simulink model "ThrottleAirMassFlow"  (R2025b)
settings: Solver=FixedStepAuto  StartTime=0.0  StopTime=200  FixedStep=0.001  RelTol=1e-3
undefined symbols (not defined in the file): R
settings Model: Creator=khanh  LastModifiedBy=khanh

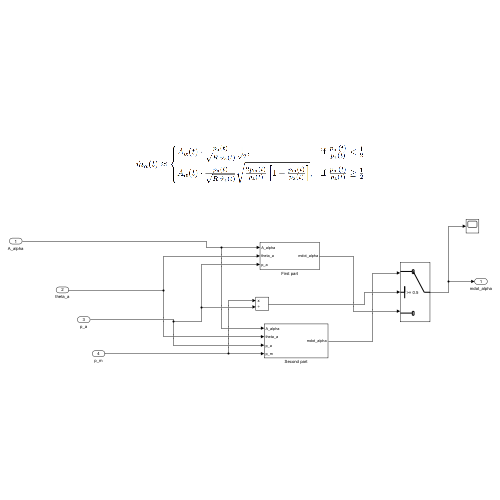
[thumbnail: Simulink's stored preview of the top-level diagram]
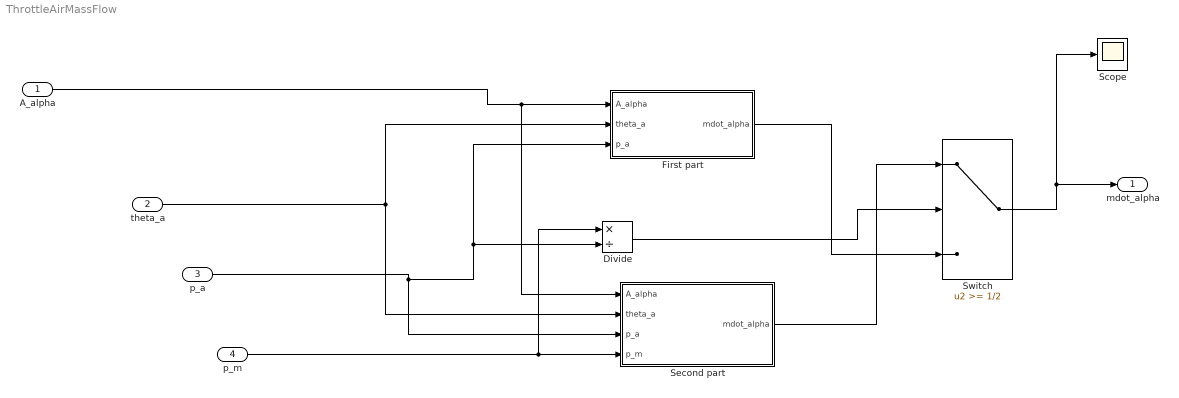
== system ThrottleAirMassFlow ==
  A_alpha : Inport
  theta_a : Inport  Port=2
  p_a : Inport  Port=3
  p_m : Inport  Port=4
  Divide : Product  Inputs=*/
  First part : Subsystem
  Scope : Scope
      settings: ActiveDisplayYMinimum=154.82054401919723  ActiveDisplayYMaximum=232.27112620786752
  "Second part " : Subsystem
  Switch : Switch  Threshold=1/2  SaturateOnIntegerOverflow=off  InputSameDT=off
  mdot_alpha : Outport
  wires:
  theta_a/1 -> "Second part "/2(theta_a), First part/2(theta_a)
  p_a/1 -> "Second part "/3(p_a), First part/3(p_a), Divide/2
  p_m/1 -> "Second part "/4(p_m), Divide/1
  Divide/1 -> Switch/2
  First part/1(mdot_alpha) -> Switch/3
  Switch/1 -> Scope/1, mdot_alpha/1
  "Second part "/1(mdot_alpha) -> Switch/1
  A_alpha/1 -> "Second part "/1(A_alpha), First part/1(A_alpha)

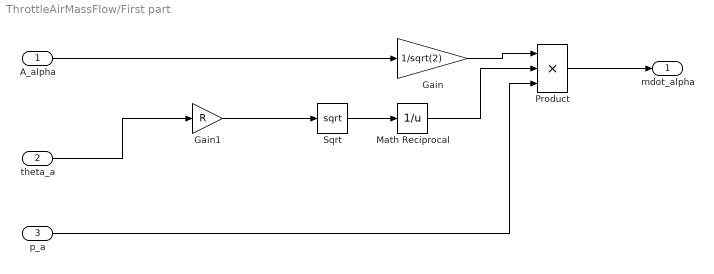
== system ThrottleAirMassFlow/First part ==
  A_alpha : Inport
  theta_a : Inport  Port=2
  p_a : Inport  Port=3
  Gain : Gain  Gain=1/sqrt(2)
  Gain1 : Gain  Gain=R
  Math Reciprocal : Math  Operator=reciprocal  SignedPower=on
  Product : Product  Inputs=3
  Sqrt : Sqrt
  mdot_alpha : Outport
  wires:
  Sqrt/1 -> Math Reciprocal/1
  p_a/1 -> Product/3
  Gain/1 -> Product/1
  Gain1/1 -> Sqrt/1
  theta_a/1 -> Gain1/1
  Product/1 -> mdot_alpha/1
  A_alpha/1 -> Gain/1
  Math Reciprocal/1 -> Product/2

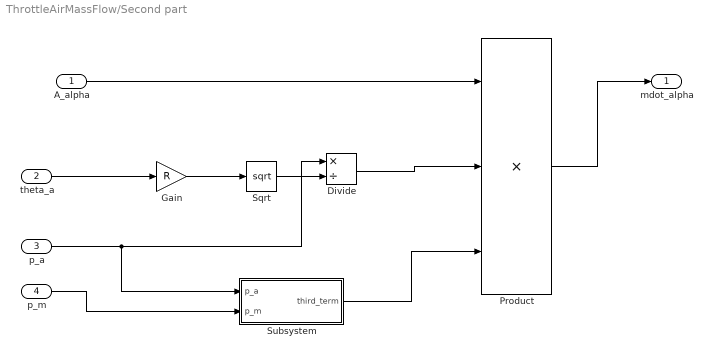
== system ThrottleAirMassFlow/Second part  ==
  A_alpha : Inport
  theta_a : Inport  Port=2
  p_a : Inport  Port=3
  p_m : Inport  Port=4
  Divide : Product  Inputs=*/
  Gain : Gain  Gain=R
  Product : Product  Inputs=3
  Sqrt : Sqrt
  Subsystem : Subsystem
  mdot_alpha : Outport
  wires:
  Product/1 -> mdot_alpha/1
  A_alpha/1 -> Product/1
  theta_a/1 -> Gain/1
  Gain/1 -> Sqrt/1
  Sqrt/1 -> Divide/2
  p_a/1 -> Subsystem/1(p_a), Divide/1
  Divide/1 -> Product/2
  p_m/1 -> Subsystem/2(p_m)
  Subsystem/1(third_term) -> Product/3

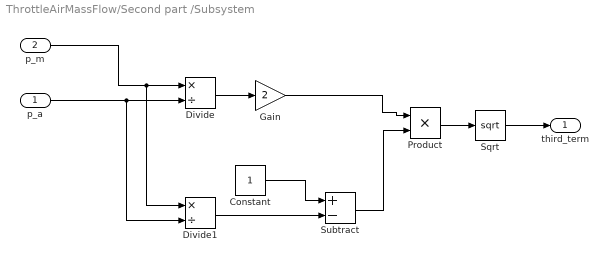
== system ThrottleAirMassFlow/Second part /Subsystem ==
  p_a : Inport
  p_m : Inport  Port=2
  Constant : Constant
  Divide : Product  Inputs=*/
  Divide1 : Product  Inputs=*/
  Gain : Gain  Gain=2
  Product : Product
  Sqrt : Sqrt
  Subtract : Sum  Inputs=+-
  third_term : Outport
  wires:
  Divide/1 -> Gain/1
  p_a/1 -> Divide1/2, Divide/2
  p_m/1 -> Divide1/1, Divide/1
  Divide1/1 -> Subtract/2
  Constant/1 -> Subtract/1
  Gain/1 -> Product/1
  Subtract/1 -> Product/2
  Product/1 -> Sqrt/1
  Sqrt/1 -> third_term/1
